simulink model "compare"  (R2015a)
settings: Solver=ode45  StartTime=0.0  StopTime=10.0  RelTol=1e-3
InitFcn:
  | %% DSPBuilder Start
  | alt_dspbuilder_update_model(bdroot)
  | %% DSPBuilder End
libraries: allblocks_alteradspbuilder2 x801
(part 1 of 9)
settings Model: Creator=ASUS  LastModifiedBy=ASUS

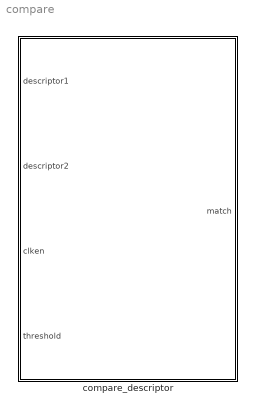
== system compare ==
  compare_descriptor : Subsystem

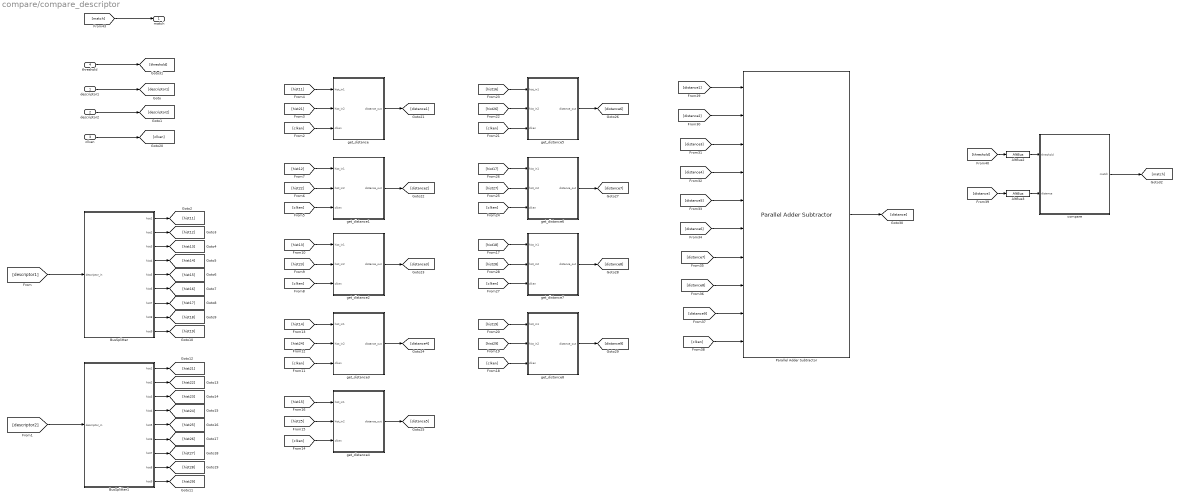
== system compare/compare_descriptor ==
  descriptor1 : Inport
  descriptor2 : Inport  Port=2
  clken : Inport  Port=3
  threshold : Inport  Port=4
  AltBus2 : allblocks_alteradspbuilder2/AltBus  BusType=Unsigned Integer  bwl=16  bwr=0  saturate=off  floatingPointInput=on  floatingPointOutput=on  logOutputs=off  logFile=C:\Users\ASUS\Desktop\final_sift_fpga\tb_compare\compare_compare%5Fdescriptor_AltBus2.fixedpointlog
  AltBus3 : allblocks_alteradspbuilder2/AltBus  BusType=Unsigned Integer  bwl=16  bwr=0  saturate=off  floatingPointInput=on  floatingPointOutput=on  logOutputs=off  logFile=C:\Users\ASUS\Desktop\final_sift_fpga\tb_compare\compare_compare%5Fdescriptor_AltBus3.fixedpointlog
  BusSplitter : Subsystem
  BusSplitter1 : Subsystem
  Parallel Adder Subtractor : allblocks_alteradspbuilder2/Parallel Adder Subtractor  number_of_inputs=9  direction=+  use_pipeline=on  pipeline_display=4  phase_selection=1  use_ena=on  use_aclr=off  allowFloatingPointOverride=on  logOutputs=off  logFile=C:\Users\ASUS\Desktop\final_sift_fpga\tb_compare\compare_compare%5Fdescriptor_Parallel+Adder+Subtractor.fixedpointlog
  compare : Subsystem
  get_distance : Subsystem
  get_distance1 : Subsystem
  get_distance2 : Subsystem
  get_distance3 : Subsystem
  get_distance4 : Subsystem
  get_distance5 : Subsystem
  get_distance6 : Subsystem
  get_distance7 : Subsystem
  get_distance8 : Subsystem
  match : Outport
  wires:
  descriptor1/1 -> [descriptor1]
  descriptor2/1 -> [descriptor2]
  [descriptor1] -> BusSplitter/1(descriptor_in)
  [descriptor2] -> BusSplitter1/1(descriptor_in)
  BusSplitter/1(hist1) -> [hist11]
  BusSplitter/2(hist2) -> [hist12]
  BusSplitter/3(hist3) -> [hist13]
  BusSplitter/4(hist4) -> [hist14]
  BusSplitter/5(hist5) -> [hist15]
  BusSplitter/6(hist6) -> [hist16]
  BusSplitter/7(hist7) -> [hist17]
  BusSplitter/8(hist8) -> [hist18]
  BusSplitter/9(hist9) -> [hist19]
  BusSplitter1/1(hist1) -> [hist21]
  BusSplitter1/2(hist2) -> [hist22]
  BusSplitter1/3(hist3) -> [hist23]
  BusSplitter1/4(hist4) -> [hist24]
  BusSplitter1/5(hist5) -> [hist25]
  BusSplitter1/6(hist6) -> [hist26]
  BusSplitter1/7(hist7) -> [hist27]
  BusSplitter1/8(hist8) -> [hist28]
  BusSplitter1/9(hist9) -> [hist29]
  clken/1 -> [clken]
  [clken] -> get_distance/3(clken)
  [hist21] -> get_distance/2(hist_in2)
  [hist11] -> get_distance/1(hist_in1)
  get_distance/1(distance_out) -> [distance1]
  [clken] -> get_distance1/3(clken)
  [hist22] -> get_distance1/2(hist_in2)
  [hist12] -> get_distance1/1(hist_in1)
  get_distance1/1(distance_out) -> [distance2]
  [clken] -> get_distance2/3(clken)
  [hist23] -> get_distance2/2(hist_in2)
  [hist13] -> get_distance2/1(hist_in1)
  get_distance2/1(distance_out) -> [distance3]
  [clken] -> get_distance3/3(clken)
  [hist24] -> get_distance3/2(hist_in2)
  [hist14] -> get_distance3/1(hist_in1)
  get_distance3/1(distance_out) -> [distance4]
  [clken] -> get_distance4/3(clken)
  [hist25] -> get_distance4/2(hist_in2)
  [hist15] -> get_distance4/1(hist_in1)
  get_distance4/1(distance_out) -> [distance5]
  [clken] -> get_distance5/3(clken)
  [hist26] -> get_distance5/2(hist_in2)
  [hist16] -> get_distance5/1(hist_in1)
  get_distance5/1(distance_out) -> [distance6]
  [clken] -> get_distance6/3(clken)
  [hist27] -> get_distance6/2(hist_in2)
  [hist17] -> get_distance6/1(hist_in1)
  get_distance6/1(distance_out) -> [distance7]
  [clken] -> get_distance7/3(clken)
  [hist28] -> get_distance7/2(hist_in2)
  [hist18] -> get_distance7/1(hist_in1)
  get_distance7/1(distance_out) -> [distance8]
  [clken] -> get_distance8/3(clken)
  [hist29] -> get_distance8/2(hist_in2)
  [hist19] -> get_distance8/1(hist_in1)
  get_distance8/1(distance_out) -> [distance9]
  [distance1] -> Parallel Adder Subtractor/1
  [distance2] -> Parallel Adder Subtractor/2
  [distance3] -> Parallel Adder Subtractor/3
  [distance4] -> Parallel Adder Subtractor/4
  [distance5] -> Parallel Adder Subtractor/5
  [distance6] -> Parallel Adder Subtractor/6
  [distance7] -> Parallel Adder Subtractor/7
  [distance8] -> Parallel Adder Subtractor/8
  [distance9] -> Parallel Adder Subtractor/9
  [clken] -> Parallel Adder Subtractor/10
  threshold/1 -> [threshold]
  [distance] -> AltBus3/1
  [threshold] -> AltBus2/1
  [match] -> match/1
  compare/1(match) -> [match]
  Parallel Adder Subtractor/1 -> [distance]
  AltBus2/1 -> compare/1(threshold)
  AltBus3/1 -> compare/2(distance)

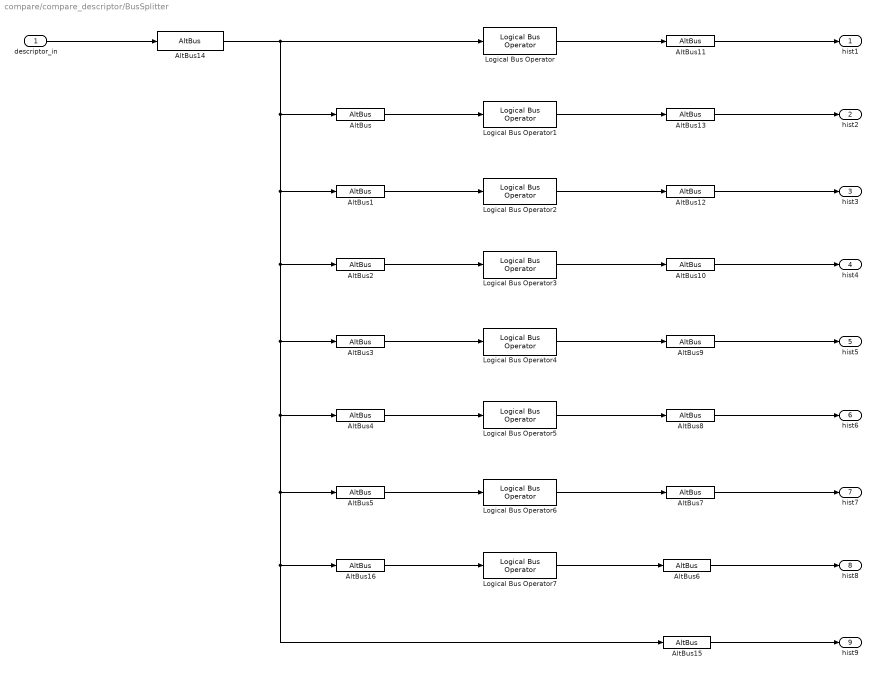
== system compare/compare_descriptor/BusSplitter ==
  descriptor_in : Inport
  AltBus : allblocks_alteradspbuilder2/AltBus  BusType=Unsigned Integer  bwl=1024  bwr=0  saturate=off  floatingPointInput=on  floatingPointOutput=on  logOutputs=off  logFile=C:\Users\ASUS\Desktop\sift_fpga\Octave_2\tb_test_final_sift\test%5Ffinal%5Fsift_sift%5Foctave1_matching_compare%5Fdescriptor_BusSplitter_AltBus.fixedpointlog
  AltBus1 : allblocks_alteradspbuilder2/AltBus  BusType=Unsigned Integer  bwl=896  bwr=0  saturate=off  floatingPointInput=on  floatingPointOutput=on  logOutputs=off  logFile=C:\Users\ASUS\Desktop\sift_fpga\Octave_2\tb_test_final_sift\test%5Ffinal%5Fsift_sift%5Foctave1_matching_compare%5Fdescriptor_BusSplitter_AltBus1.fixedpointlog
  AltBus10 : allblocks_alteradspbuilder2/AltBus  BusType=Unsigned Integer  bwl=128  bwr=0  saturate=off  floatingPointInput=on  floatingPointOutput=on  logOutputs=off  logFile=C:\Users\ASUS\Desktop\sift_fpga\Octave_2\tb_test_final_sift\test%5Ffinal%5Fsift_sift%5Foctave1_matching_compare%5Fdescriptor_BusSplitter_AltBus10.fixedpointlog
  AltBus11 : allblocks_alteradspbuilder2/AltBus  BusType=Unsigned Integer  bwl=128  bwr=0  saturate=off  floatingPointInput=on  floatingPointOutput=on  logOutputs=off  logFile=C:\Users\ASUS\Desktop\sift_fpga\Octave_2\tb_test_final_sift\test%5Ffinal%5Fsift_sift%5Foctave1_matching_compare%5Fdescriptor_BusSplitter_AltBus11.fixedpointlog
  AltBus12 : allblocks_alteradspbuilder2/AltBus  BusType=Unsigned Integer  bwl=128  bwr=0  saturate=off  floatingPointInput=on  floatingPointOutput=on  logOutputs=off  logFile=C:\Users\ASUS\Desktop\sift_fpga\Octave_2\tb_test_final_sift\test%5Ffinal%5Fsift_sift%5Foctave1_matching_compare%5Fdescriptor_BusSplitter_AltBus12.fixedpointlog
  AltBus13 : allblocks_alteradspbuilder2/AltBus  BusType=Unsigned Integer  bwl=128  bwr=0  saturate=off  floatingPointInput=on  floatingPointOutput=on  logOutputs=off  logFile=C:\Users\ASUS\Desktop\sift_fpga\Octave_2\tb_test_final_sift\test%5Ffinal%5Fsift_sift%5Foctave1_matching_compare%5Fdescriptor_BusSplitter_AltBus13.fixedpointlog
  AltBus14 : allblocks_alteradspbuilder2/AltBus  BusType=Unsigned Integer  bwl=16*8*9  bwr=0  saturate=off  floatingPointInput=on  floatingPointOutput=on  logOutputs=off  logFile=C:\Users\ASUS\Desktop\sift_fpga\Octave_2\tb_test_final_sift\test%5Ffinal%5Fsift_sift%5Foctave1_matching_compare%5Fdescriptor_BusSplitter_AltBus14.fixedpointlog
  AltBus15 : allblocks_alteradspbuilder2/AltBus  BusType=Unsigned Integer  bwl=128  bwr=0  saturate=off  floatingPointInput=on  floatingPointOutput=on  logOutputs=off  logFile=C:\Users\ASUS\Desktop\sift_fpga\Octave_2\tb_test_final_sift\test%5Ffinal%5Fsift_sift%5Foctave1_matching_compare%5Fdescriptor_BusSplitter_AltBus15.fixedpointlog
  AltBus16 : allblocks_alteradspbuilder2/AltBus  BusType=Unsigned Integer  bwl=256  bwr=0  saturate=off  floatingPointInput=on  floatingPointOutput=on  logOutputs=off  logFile=C:\Users\ASUS\Desktop\sift_fpga\Octave_2\tb_test_final_sift\test%5Ffinal%5Fsift_sift%5Foctave1_matching_compare%5Fdescriptor_BusSplitter_AltBus16.fixedpointlog
  AltBus2 : allblocks_alteradspbuilder2/AltBus  BusType=Unsigned Integer  bwl=768  bwr=0  saturate=off  floatingPointInput=on  floatingPointOutput=on  logOutputs=off  logFile=C:\Users\ASUS\Desktop\sift_fpga\Octave_2\tb_test_final_sift\test%5Ffinal%5Fsift_sift%5Foctave1_matching_compare%5Fdescriptor_BusSplitter_AltBus2.fixedpointlog
  AltBus3 : allblocks_alteradspbuilder2/AltBus  BusType=Unsigned Integer  bwl=640  bwr=0  saturate=off  floatingPointInput=on  floatingPointOutput=on  logOutputs=off  logFile=C:\Users\ASUS\Desktop\sift_fpga\Octave_2\tb_test_final_sift\test%5Ffinal%5Fsift_sift%5Foctave1_matching_compare%5Fdescriptor_BusSplitter_AltBus3.fixedpointlog
  AltBus4 : allblocks_alteradspbuilder2/AltBus  BusType=Unsigned Integer  bwl=512  bwr=0  saturate=off  floatingPointInput=on  floatingPointOutput=on  logOutputs=off  logFile=C:\Users\ASUS\Desktop\sift_fpga\Octave_2\tb_test_final_sift\test%5Ffinal%5Fsift_sift%5Foctave1_matching_compare%5Fdescriptor_BusSplitter_AltBus4.fixedpointlog
  AltBus5 : allblocks_alteradspbuilder2/AltBus  BusType=Unsigned Integer  bwl=384  bwr=0  saturate=off  floatingPointInput=on  floatingPointOutput=on  logOutputs=off  logFile=C:\Users\ASUS\Desktop\sift_fpga\Octave_2\tb_test_final_sift\test%5Ffinal%5Fsift_sift%5Foctave1_matching_compare%5Fdescriptor_BusSplitter_AltBus5.fixedpointlog
  AltBus6 : allblocks_alteradspbuilder2/AltBus  BusType=Unsigned Integer  bwl=128  bwr=0  saturate=off  floatingPointInput=on  floatingPointOutput=on  logOutputs=off  logFile=C:\Users\ASUS\Desktop\sift_fpga\Octave_2\tb_test_final_sift\test%5Ffinal%5Fsift_sift%5Foctave1_matching_compare%5Fdescriptor_BusSplitter_AltBus6.fixedpointlog
  AltBus7 : allblocks_alteradspbuilder2/AltBus  BusType=Unsigned Integer  bwl=128  bwr=0  saturate=off  floatingPointInput=on  floatingPointOutput=on  logOutputs=off  logFile=C:\Users\ASUS\Desktop\sift_fpga\Octave_2\tb_test_final_sift\test%5Ffinal%5Fsift_sift%5Foctave1_matching_compare%5Fdescriptor_BusSplitter_AltBus7.fixedpointlog
  AltBus8 : allblocks_alteradspbuilder2/AltBus  BusType=Unsigned Integer  bwl=128  bwr=0  saturate=off  floatingPointInput=on  floatingPointOutput=on  logOutputs=off  logFile=C:\Users\ASUS\Desktop\sift_fpga\Octave_2\tb_test_final_sift\test%5Ffinal%5Fsift_sift%5Foctave1_matching_compare%5Fdescriptor_BusSplitter_AltBus8.fixedpointlog
  AltBus9 : allblocks_alteradspbuilder2/AltBus  BusType=Unsigned Integer  bwl=128  bwr=0  saturate=off  floatingPointInput=on  floatingPointOutput=on  logOutputs=off  logFile=C:\Users\ASUS\Desktop\sift_fpga\Octave_2\tb_test_final_sift\test%5Ffinal%5Fsift_sift%5Foctave1_matching_compare%5Fdescriptor_BusSplitter_AltBus9.fixedpointlog
  Logical Bus Operator : allblocks_alteradspbuilder2/Logical Bus Operator  BusType=Unsigned Integer  bwl=1152  bwr=0  LogicalOp_text=Shift Right  mask_value_num=-5  shift_amount=8*128  force_sign_ext=off  pipeline_display=0
  Logical Bus Operator1 : allblocks_alteradspbuilder2/Logical Bus Operator  BusType=Unsigned Integer  bwl=1024  bwr=0  LogicalOp_text=Shift Right  mask_value_num=-5  shift_amount=7*128  force_sign_ext=off  pipeline_display=0
  Logical Bus Operator2 : allblocks_alteradspbuilder2/Logical Bus Operator  BusType=Unsigned Integer  bwl=896  bwr=0  LogicalOp_text=Shift Right  mask_value_num=-5  shift_amount=6*128  force_sign_ext=off  pipeline_display=0
  Logical Bus Operator3 : allblocks_alteradspbuilder2/Logical Bus Operator  BusType=Unsigned Integer  bwl=768  bwr=0  LogicalOp_text=Shift Right  mask_value_num=-5  shift_amount=5*128  force_sign_ext=off  pipeline_display=0
  Logical Bus Operator4 : allblocks_alteradspbuilder2/Logical Bus Operator  BusType=Unsigned Integer  bwl=640  bwr=0  LogicalOp_text=Shift Right  mask_value_num=-5  shift_amount=4*128  force_sign_ext=off  pipeline_display=0
  Logical Bus Operator5 : allblocks_alteradspbuilder2/Logical Bus Operator  BusType=Unsigned Integer  bwl=512  bwr=0  LogicalOp_text=Shift Right  mask_value_num=-5  shift_amount=3*128  force_sign_ext=off  pipeline_display=0
  Logical Bus Operator6 : allblocks_alteradspbuilder2/Logical Bus Operator  BusType=Unsigned Integer  bwl=384  bwr=0  LogicalOp_text=Shift Right  mask_value_num=-5  shift_amount=2*128  force_sign_ext=off  pipeline_display=0
  Logical Bus Operator7 : allblocks_alteradspbuilder2/Logical Bus Operator  BusType=Unsigned Integer  bwl=256  bwr=0  LogicalOp_text=Shift Right  mask_value_num=-5  shift_amount=128  force_sign_ext=off  pipeline_display=0
  hist1 : Outport
  hist2 : Outport  Port=2
  hist3 : Outport  Port=3
  hist4 : Outport  Port=4
  hist5 : Outport  Port=5
  hist6 : Outport  Port=6
  hist7 : Outport  Port=7
  hist8 : Outport  Port=8
  hist9 : Outport  Port=9
  wires:
  Logical Bus Operator6/1 -> AltBus7/1
  AltBus1/1 -> Logical Bus Operator2/1
  AltBus9/1 -> hist5/1
  AltBus8/1 -> hist6/1
  AltBus7/1 -> hist7/1
  AltBus6/1 -> hist8/1
  AltBus/1 -> Logical Bus Operator1/1
  AltBus10/1 -> hist4/1
  AltBus12/1 -> hist3/1
  AltBus11/1 -> hist1/1
  AltBus3/1 -> Logical Bus Operator4/1
  AltBus2/1 -> Logical Bus Operator3/1
  AltBus4/1 -> Logical Bus Operator5/1
  descriptor_in/1 -> AltBus14/1
  AltBus5/1 -> Logical Bus Operator6/1
  Logical Bus Operator1/1 -> AltBus13/1
  Logical Bus Operator2/1 -> AltBus12/1
  Logical Bus Operator/1 -> AltBus11/1
  Logical Bus Operator5/1 -> AltBus8/1
  Logical Bus Operator4/1 -> AltBus9/1
  Logical Bus Operator3/1 -> AltBus10/1
  AltBus13/1 -> hist2/1
  AltBus15/1 -> hist9/1
  AltBus14/1 -> AltBus15/1, AltBus16/1, AltBus5/1, AltBus4/1, AltBus3/1, AltBus2/1, AltBus1/1, AltBus/1, Logical Bus Operator/1
  AltBus16/1 -> Logical Bus Operator7/1
  Logical Bus Operator7/1 -> AltBus6/1

== system compare/compare_descriptor/BusSplitter1 ==
  descriptor_in : Inport
  AltBus : allblocks_alteradspbuilder2/AltBus  BusType=Unsigned Integer  bwl=1024  bwr=0  saturate=off  floatingPointInput=on  floatingPointOutput=on  logOutputs=off  logFile=C:\Users\ASUS\Desktop\sift_fpga\Octave_2\tb_test_final_sift\test%5Ffinal%5Fsift_sift%5Foctave1_matching_compare%5Fdescriptor_BusSplitter1_AltBus.fixedpointlog
  AltBus1 : allblocks_alteradspbuilder2/AltBus  BusType=Unsigned Integer  bwl=896  bwr=0  saturate=off  floatingPointInput=on  floatingPointOutput=on  logOutputs=off  logFile=C:\Users\ASUS\Desktop\sift_fpga\Octave_2\tb_test_final_sift\test%5Ffinal%5Fsift_sift%5Foctave1_matching_compare%5Fdescriptor_BusSplitter1_AltBus1.fixedpointlog
  AltBus10 : allblocks_alteradspbuilder2/AltBus  BusType=Unsigned Integer  bwl=128  bwr=0  saturate=off  floatingPointInput=on  floatingPointOutput=on  logOutputs=off  logFile=C:\Users\ASUS\Desktop\sift_fpga\Octave_2\tb_test_final_sift\test%5Ffinal%5Fsift_sift%5Foctave1_matching_compare%5Fdescriptor_BusSplitter1_AltBus10.fixedpointlog
  AltBus11 : allblocks_alteradspbuilder2/AltBus  BusType=Unsigned Integer  bwl=128  bwr=0  saturate=off  floatingPointInput=on  floatingPointOutput=on  logOutputs=off  logFile=C:\Users\ASUS\Desktop\sift_fpga\Octave_2\tb_test_final_sift\test%5Ffinal%5Fsift_sift%5Foctave1_matching_compare%5Fdescriptor_BusSplitter1_AltBus11.fixedpointlog
  AltBus12 : allblocks_alteradspbuilder2/AltBus  BusType=Unsigned Integer  bwl=128  bwr=0  saturate=off  floatingPointInput=on  floatingPointOutput=on  logOutputs=off  logFile=C:\Users\ASUS\Desktop\sift_fpga\Octave_2\tb_test_final_sift\test%5Ffinal%5Fsift_sift%5Foctave1_matching_compare%5Fdescriptor_BusSplitter1_AltBus12.fixedpointlog
  AltBus13 : allblocks_alteradspbuilder2/AltBus  BusType=Unsigned Integer  bwl=128  bwr=0  saturate=off  floatingPointInput=on  floatingPointOutput=on  logOutputs=off  logFile=C:\Users\ASUS\Desktop\sift_fpga\Octave_2\tb_test_final_sift\test%5Ffinal%5Fsift_sift%5Foctave1_matching_compare%5Fdescriptor_BusSplitter1_AltBus13.fixedpointlog
  AltBus14 : allblocks_alteradspbuilder2/AltBus  BusType=Unsigned Integer  bwl=16*8*9  bwr=0  saturate=off  floatingPointInput=on  floatingPointOutput=on  logOutputs=off  logFile=C:\Users\ASUS\Desktop\sift_fpga\Octave_2\tb_test_final_sift\test%5Ffinal%5Fsift_sift%5Foctave1_matching_compare%5Fdescriptor_BusSplitter1_AltBus14.fixedpointlog
  AltBus15 : allblocks_alteradspbuilder2/AltBus  BusType=Unsigned Integer  bwl=128  bwr=0  saturate=off  floatingPointInput=on  floatingPointOutput=on  logOutputs=off  logFile=C:\Users\ASUS\Desktop\sift_fpga\Octave_2\tb_test_final_sift\test%5Ffinal%5Fsift_sift%5Foctave1_matching_compare%5Fdescriptor_BusSplitter1_AltBus15.fixedpointlog
  AltBus16 : allblocks_alteradspbuilder2/AltBus  BusType=Unsigned Integer  bwl=256  bwr=0  saturate=off  floatingPointInput=on  floatingPointOutput=on  logOutputs=off  logFile=C:\Users\ASUS\Desktop\sift_fpga\Octave_2\tb_test_final_sift\test%5Ffinal%5Fsift_sift%5Foctave1_matching_compare%5Fdescriptor_BusSplitter1_AltBus16.fixedpointlog
  AltBus2 : allblocks_alteradspbuilder2/AltBus  BusType=Unsigned Integer  bwl=768  bwr=0  saturate=off  floatingPointInput=on  floatingPointOutput=on  logOutputs=off  logFile=C:\Users\ASUS\Desktop\sift_fpga\Octave_2\tb_test_final_sift\test%5Ffinal%5Fsift_sift%5Foctave1_matching_compare%5Fdescriptor_BusSplitter1_AltBus2.fixedpointlog
  AltBus3 : allblocks_alteradspbuilder2/AltBus  BusType=Unsigned Integer  bwl=640  bwr=0  saturate=off  floatingPointInput=on  floatingPointOutput=on  logOutputs=off  logFile=C:\Users\ASUS\Desktop\sift_fpga\Octave_2\tb_test_final_sift\test%5Ffinal%5Fsift_sift%5Foctave1_matching_compare%5Fdescriptor_BusSplitter1_AltBus3.fixedpointlog
  AltBus4 : allblocks_alteradspbuilder2/AltBus  BusType=Unsigned Integer  bwl=512  bwr=0  saturate=off  floatingPointInput=on  floatingPointOutput=on  logOutputs=off  logFile=C:\Users\ASUS\Desktop\sift_fpga\Octave_2\tb_test_final_sift\test%5Ffinal%5Fsift_sift%5Foctave1_matching_compare%5Fdescriptor_BusSplitter1_AltBus4.fixedpointlog
  AltBus5 : allblocks_alteradspbuilder2/AltBus  BusType=Unsigned Integer  bwl=384  bwr=0  saturate=off  floatingPointInput=on  floatingPointOutput=on  logOutputs=off  logFile=C:\Users\ASUS\Desktop\sift_fpga\Octave_2\tb_test_final_sift\test%5Ffinal%5Fsift_sift%5Foctave1_matching_compare%5Fdescriptor_BusSplitter1_AltBus5.fixedpointlog
  AltBus6 : allblocks_alteradspbuilder2/AltBus  BusType=Unsigned Integer  bwl=128  bwr=0  saturate=off  floatingPointInput=on  floatingPointOutput=on  logOutputs=off  logFile=C:\Users\ASUS\Desktop\sift_fpga\Octave_2\tb_test_final_sift\test%5Ffinal%5Fsift_sift%5Foctave1_matching_compare%5Fdescriptor_BusSplitter1_AltBus6.fixedpointlog
  AltBus7 : allblocks_alteradspbuilder2/AltBus  BusType=Unsigned Integer  bwl=128  bwr=0  saturate=off  floatingPointInput=on  floatingPointOutput=on  logOutputs=off  logFile=C:\Users\ASUS\Desktop\sift_fpga\Octave_2\tb_test_final_sift\test%5Ffinal%5Fsift_sift%5Foctave1_matching_compare%5Fdescriptor_BusSplitter1_AltBus7.fixedpointlog
  AltBus8 : allblocks_alteradspbuilder2/AltBus  BusType=Unsigned Integer  bwl=128  bwr=0  saturate=off  floatingPointInput=on  floatingPointOutput=on  logOutputs=off  logFile=C:\Users\ASUS\Desktop\sift_fpga\Octave_2\tb_test_final_sift\test%5Ffinal%5Fsift_sift%5Foctave1_matching_compare%5Fdescriptor_BusSplitter1_AltBus8.fixedpointlog
  AltBus9 : allblocks_alteradspbuilder2/AltBus  BusType=Unsigned Integer  bwl=128  bwr=0  saturate=off  floatingPointInput=on  floatingPointOutput=on  logOutputs=off  logFile=C:\Users\ASUS\Desktop\sift_fpga\Octave_2\tb_test_final_sift\test%5Ffinal%5Fsift_sift%5Foctave1_matching_compare%5Fdescriptor_BusSplitter1_AltBus9.fixedpointlog
  Logical Bus Operator : allblocks_alteradspbuilder2/Logical Bus Operator  BusType=Unsigned Integer  bwl=1152  bwr=0  LogicalOp_text=Shift Right  mask_value_num=-5  shift_amount=8*128  force_sign_ext=off  pipeline_display=0
  Logical Bus Operator1 : allblocks_alteradspbuilder2/Logical Bus Operator  BusType=Unsigned Integer  bwl=1024  bwr=0  LogicalOp_text=Shift Right  mask_value_num=-5  shift_amount=7*128  force_sign_ext=off  pipeline_display=0
  Logical Bus Operator2 : allblocks_alteradspbuilder2/Logical Bus Operator  BusType=Unsigned Integer  bwl=896  bwr=0  LogicalOp_text=Shift Right  mask_value_num=-5  shift_amount=6*128  force_sign_ext=off  pipeline_display=0
  Logical Bus Operator3 : allblocks_alteradspbuilder2/Logical Bus Operator  BusType=Unsigned Integer  bwl=768  bwr=0  LogicalOp_text=Shift Right  mask_value_num=-5  shift_amount=5*128  force_sign_ext=off  pipeline_display=0
  Logical Bus Operator4 : allblocks_alteradspbuilder2/Logical Bus Operator  BusType=Unsigned Integer  bwl=640  bwr=0  LogicalOp_text=Shift Right  mask_value_num=-5  shift_amount=4*128  force_sign_ext=off  pipeline_display=0
  Logical Bus Operator5 : allblocks_alteradspbuilder2/Logical Bus Operator  BusType=Unsigned Integer  bwl=512  bwr=0  LogicalOp_text=Shift Right  mask_value_num=-5  shift_amount=3*128  force_sign_ext=off  pipeline_display=0
  Logical Bus Operator6 : allblocks_alteradspbuilder2/Logical Bus Operator  BusType=Unsigned Integer  bwl=384  bwr=0  LogicalOp_text=Shift Right  mask_value_num=-5  shift_amount=2*128  force_sign_ext=off  pipeline_display=0
  Logical Bus Operator7 : allblocks_alteradspbuilder2/Logical Bus Operator  BusType=Unsigned Integer  bwl=256  bwr=0  LogicalOp_text=Shift Right  mask_value_num=-5  shift_amount=128  force_sign_ext=off  pipeline_display=0
  hist1 : Outport
  hist2 : Outport  Port=2
  hist3 : Outport  Port=3
  hist4 : Outport  Port=4
  hist5 : Outport  Port=5
  hist6 : Outport  Port=6
  hist7 : Outport  Port=7
  hist8 : Outport  Port=8
  hist9 : Outport  Port=9
  wires:
  Logical Bus Operator6/1 -> AltBus7/1
  AltBus1/1 -> Logical Bus Operator2/1
  AltBus9/1 -> hist5/1
  AltBus8/1 -> hist6/1
  AltBus7/1 -> hist7/1
  AltBus6/1 -> hist8/1
  AltBus/1 -> Logical Bus Operator1/1
  AltBus10/1 -> hist4/1
  AltBus12/1 -> hist3/1
  AltBus11/1 -> hist1/1
  AltBus3/1 -> Logical Bus Operator4/1
  AltBus2/1 -> Logical Bus Operator3/1
  AltBus4/1 -> Logical Bus Operator5/1
  descriptor_in/1 -> AltBus14/1
  AltBus5/1 -> Logical Bus Operator6/1
  Logical Bus Operator1/1 -> AltBus13/1
  Logical Bus Operator2/1 -> AltBus12/1
  Logical Bus Operator/1 -> AltBus11/1
  Logical Bus Operator5/1 -> AltBus8/1
  Logical Bus Operator4/1 -> AltBus9/1
  Logical Bus Operator3/1 -> AltBus10/1
  AltBus13/1 -> hist2/1
  AltBus15/1 -> hist9/1
  AltBus14/1 -> AltBus15/1, AltBus16/1, AltBus5/1, AltBus4/1, AltBus3/1, AltBus2/1, AltBus1/1, AltBus/1, Logical Bus Operator/1
  AltBus16/1 -> Logical Bus Operator7/1
  Logical Bus Operator7/1 -> AltBus6/1

== system compare/compare_descriptor/compare ==
  threshold : Inport
  distance : Inport  Port=2
  Comparator : allblocks_alteradspbuilder2/Comparator  direction=a > b  pipeline_display=0  allowFloatingPointOverride=on  logOutputs=off  logFile=C:\Users\ASUS\Desktop\sift_fpga\Octave_2\tb_test_final_sift\test%5Ffinal%5Fsift_sift%5Foctave1_matching_compare%5Fdescriptor_compare_Comparator.fixedpointlog
  match : Outport
  wires:
  threshold/1 -> [threshold]
  distance/1 -> [distance]
  [match] -> match/1
  [threshold] -> Comparator/1
  [distance] -> Comparator/2
  Comparator/1 -> [match]

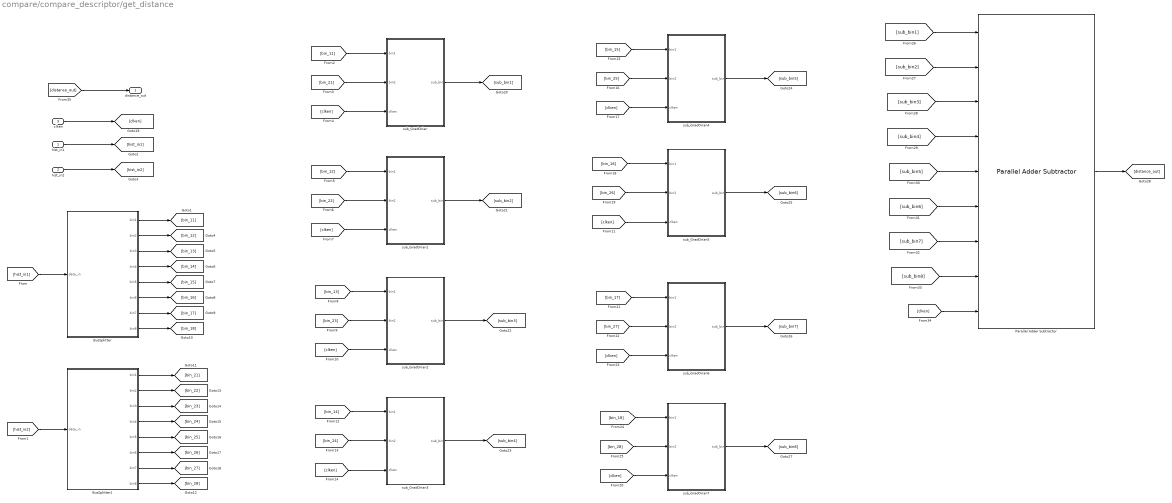
== system compare/compare_descriptor/get_distance ==
  hist_in1 : Inport
  hist_in2 : Inport  Port=2
  clken : Inport  Port=3
  BusSplitter : Subsystem
  BusSplitter1 : Subsystem
  Parallel Adder Subtractor : allblocks_alteradspbuilder2/Parallel Adder Subtractor  number_of_inputs=8  direction=+  use_pipeline=on  pipeline_display=3  phase_selection=1  use_ena=on  use_aclr=off  allowFloatingPointOverride=on  logOutputs=off  logFile=C:\Users\ASUS\Desktop\sift_fpga\Octave_2\tb_test_final_sift\test%5Ffinal%5Fsift_sift%5Foctave1_matching_compare%5Fdescriptor_get%5Fdistance_Parallel+Adder+Subtractor.fixedpointlog
  sub_GradOrian : Subsystem
  sub_GradOrian1 : Subsystem
  sub_GradOrian2 : Subsystem
  sub_GradOrian3 : Subsystem
  sub_GradOrian4 : Subsystem
  sub_GradOrian5 : Subsystem
  sub_GradOrian6 : Subsystem
  sub_GradOrian7 : Subsystem
  distance_out : Outport
  wires:
  hist_in2/1 -> [hist_in2]
  hist_in1/1 -> [hist_in1]
  [hist_in1] -> BusSplitter/1(data_in)
  [hist_in2] -> BusSplitter1/1(data_in)
  BusSplitter/1(bin1) -> [bin_11]
  BusSplitter/2(bin2) -> [bin_12]
  BusSplitter/3(bin3) -> [bin_13]
  BusSplitter/4(bin4) -> [bin_14]
  BusSplitter/5(bin5) -> [bin_15]
  BusSplitter/6(bin6) -> [bin_16]
  BusSplitter/7(bin7) -> [bin_17]
  BusSplitter/8(bin8) -> [bin_18]
  BusSplitter1/1(bin1) -> [bin_21]
  BusSplitter1/2(bin2) -> [bin_22]
  BusSplitter1/3(bin3) -> [bin_23]
  BusSplitter1/4(bin4) -> [bin_24]
  BusSplitter1/5(bin5) -> [bin_25]
  BusSplitter1/6(bin6) -> [bin_26]
  BusSplitter1/7(bin7) -> [bin_27]
  BusSplitter1/8(bin8) -> [bin_28]
  [bin_21] -> sub_GradOrian/2(bin2)
  [bin_11] -> sub_GradOrian/1(bin1)
  clken/1 -> [clken]
  [clken] -> sub_GradOrian/3(clken)
  sub_GradOrian/1(sub_bin) -> [sub_bin1]
  [bin_22] -> sub_GradOrian1/2(bin2)
  [bin_12] -> sub_GradOrian1/1(bin1)
  [clken] -> sub_GradOrian1/3(clken)
  sub_GradOrian1/1(sub_bin) -> [sub_bin2]
  [bin_23] -> sub_GradOrian2/2(bin2)
  [bin_13] -> sub_GradOrian2/1(bin1)
  [clken] -> sub_GradOrian2/3(clken)
  sub_GradOrian2/1(sub_bin) -> [sub_bin3]
  [bin_24] -> sub_GradOrian3/2(bin2)
  [bin_14] -> sub_GradOrian3/1(bin1)
  [clken] -> sub_GradOrian3/3(clken)
  sub_GradOrian3/1(sub_bin) -> [sub_bin4]
  [bin_25] -> sub_GradOrian4/2(bin2)
  [bin_15] -> sub_GradOrian4/1(bin1)
  [clken] -> sub_GradOrian4/3(clken)
  sub_GradOrian4/1(sub_bin) -> [sub_bin5]
  [bin_26] -> sub_GradOrian5/2(bin2)
  [bin_16] -> sub_GradOrian5/1(bin1)
  [clken] -> sub_GradOrian5/3(clken)
  sub_GradOrian5/1(sub_bin) -> [sub_bin6]
  [bin_27] -> sub_GradOrian6/2(bin2)
  [bin_17] -> sub_GradOrian6/1(bin1)
  [clken] -> sub_GradOrian6/3(clken)
  sub_GradOrian6/1(sub_bin) -> [sub_bin7]
  [bin_28] -> sub_GradOrian7/2(bin2)
  [bin_18] -> sub_GradOrian7/1(bin1)
  [clken] -> sub_GradOrian7/3(clken)
  sub_GradOrian7/1(sub_bin) -> [sub_bin8]
  [sub_bin1] -> Parallel Adder Subtractor/1
  [sub_bin2] -> Parallel Adder Subtractor/2
  [sub_bin3] -> Parallel Adder Subtractor/3
  [sub_bin4] -> Parallel Adder Subtractor/4
  [sub_bin5] -> Parallel Adder Subtractor/5
  [sub_bin6] -> Parallel Adder Subtractor/6
  [sub_bin7] -> Parallel Adder Subtractor/7
  [sub_bin8] -> Parallel Adder Subtractor/8
  [clken] -> Parallel Adder Subtractor/9
  Parallel Adder Subtractor/1 -> [distance_out]
  [distance_out] -> distance_out/1

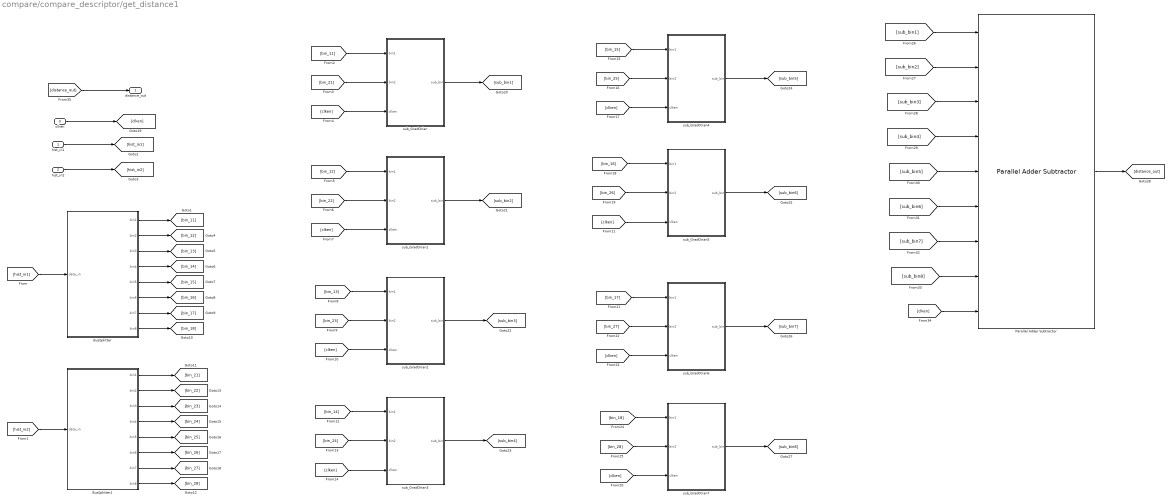
== system compare/compare_descriptor/get_distance1 ==
  hist_in1 : Inport
  hist_in2 : Inport  Port=2
  clken : Inport  Port=3
  BusSplitter : Subsystem
  BusSplitter1 : Subsystem
  Parallel Adder Subtractor : allblocks_alteradspbuilder2/Parallel Adder Subtractor  number_of_inputs=8  direction=+  use_pipeline=on  pipeline_display=3  phase_selection=1  use_ena=on  use_aclr=off  allowFloatingPointOverride=on  logOutputs=off  logFile=C:\Users\ASUS\Desktop\sift_fpga\Octave_2\tb_test_final_sift\test%5Ffinal%5Fsift_sift%5Foctave1_matching_compare%5Fdescriptor_get%5Fdistance1_Parallel+Adder+Subtractor.fixedpointlog
  sub_GradOrian : Subsystem
  sub_GradOrian1 : Subsystem
  sub_GradOrian2 : Subsystem
  sub_GradOrian3 : Subsystem
  sub_GradOrian4 : Subsystem
  sub_GradOrian5 : Subsystem
  sub_GradOrian6 : Subsystem
  sub_GradOrian7 : Subsystem
  distance_out : Outport
  wires:
  hist_in2/1 -> [hist_in2]
  hist_in1/1 -> [hist_in1]
  [hist_in1] -> BusSplitter/1(data_in)
  [hist_in2] -> BusSplitter1/1(data_in)
  BusSplitter/1(bin1) -> [bin_11]
  BusSplitter/2(bin2) -> [bin_12]
  BusSplitter/3(bin3) -> [bin_13]
  BusSplitter/4(bin4) -> [bin_14]
  BusSplitter/5(bin5) -> [bin_15]
  BusSplitter/6(bin6) -> [bin_16]
  BusSplitter/7(bin7) -> [bin_17]
  BusSplitter/8(bin8) -> [bin_18]
  BusSplitter1/1(bin1) -> [bin_21]
  BusSplitter1/2(bin2) -> [bin_22]
  BusSplitter1/3(bin3) -> [bin_23]
  BusSplitter1/4(bin4) -> [bin_24]
  BusSplitter1/5(bin5) -> [bin_25]
  BusSplitter1/6(bin6) -> [bin_26]
  BusSplitter1/7(bin7) -> [bin_27]
  BusSplitter1/8(bin8) -> [bin_28]
  [bin_21] -> sub_GradOrian/2(bin2)
  [bin_11] -> sub_GradOrian/1(bin1)
  clken/1 -> [clken]
  [clken] -> sub_GradOrian/3(clken)
  sub_GradOrian/1(sub_bin) -> [sub_bin1]
  [bin_22] -> sub_GradOrian1/2(bin2)
  [bin_12] -> sub_GradOrian1/1(bin1)
  [clken] -> sub_GradOrian1/3(clken)
  sub_GradOrian1/1(sub_bin) -> [sub_bin2]
  [bin_23] -> sub_GradOrian2/2(bin2)
  [bin_13] -> sub_GradOrian2/1(bin1)
  [clken] -> sub_GradOrian2/3(clken)
  sub_GradOrian2/1(sub_bin) -> [sub_bin3]
  [bin_24] -> sub_GradOrian3/2(bin2)
  [bin_14] -> sub_GradOrian3/1(bin1)
  [clken] -> sub_GradOrian3/3(clken)
  sub_GradOrian3/1(sub_bin) -> [sub_bin4]
  [bin_25] -> sub_GradOrian4/2(bin2)
  [bin_15] -> sub_GradOrian4/1(bin1)
  [clken] -> sub_GradOrian4/3(clken)
  sub_GradOrian4/1(sub_bin) -> [sub_bin5]
  [bin_26] -> sub_GradOrian5/2(bin2)
  [bin_16] -> sub_GradOrian5/1(bin1)
  [clken] -> sub_GradOrian5/3(clken)
  sub_GradOrian5/1(sub_bin) -> [sub_bin6]
  [bin_27] -> sub_GradOrian6/2(bin2)
  [bin_17] -> sub_GradOrian6/1(bin1)
  [clken] -> sub_GradOrian6/3(clken)
  sub_GradOrian6/1(sub_bin) -> [sub_bin7]
  [bin_28] -> sub_GradOrian7/2(bin2)
  [bin_18] -> sub_GradOrian7/1(bin1)
  [clken] -> sub_GradOrian7/3(clken)
  sub_GradOrian7/1(sub_bin) -> [sub_bin8]
  [sub_bin1] -> Parallel Adder Subtractor/1
  [sub_bin2] -> Parallel Adder Subtractor/2
  [sub_bin3] -> Parallel Adder Subtractor/3
  [sub_bin4] -> Parallel Adder Subtractor/4
  [sub_bin5] -> Parallel Adder Subtractor/5
  [sub_bin6] -> Parallel Adder Subtractor/6
  [sub_bin7] -> Parallel Adder Subtractor/7
  [sub_bin8] -> Parallel Adder Subtractor/8
  [clken] -> Parallel Adder Subtractor/9
  Parallel Adder Subtractor/1 -> [distance_out]
  [distance_out] -> distance_out/1

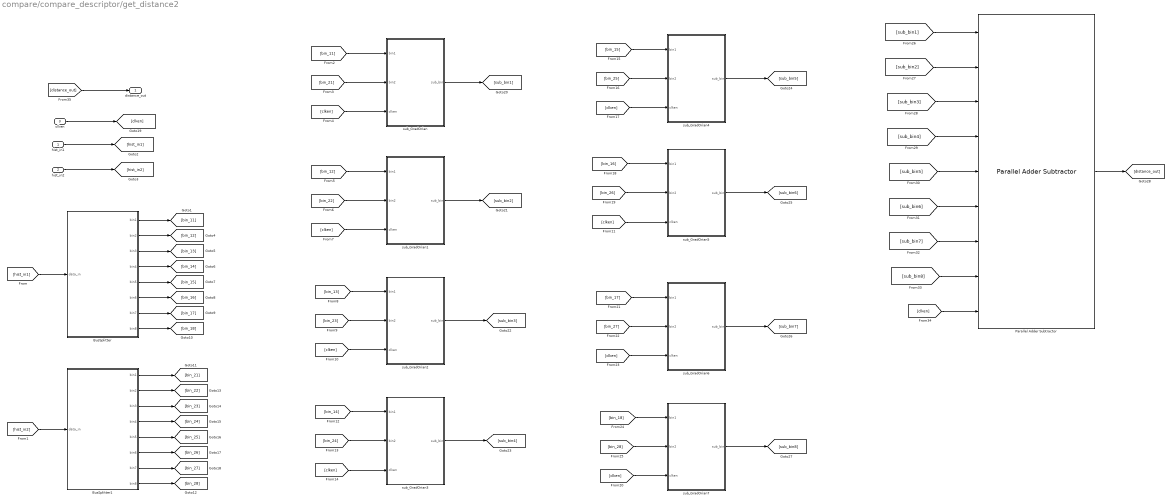
== system compare/compare_descriptor/get_distance2 ==
  hist_in1 : Inport
  hist_in2 : Inport  Port=2
  clken : Inport  Port=3
  BusSplitter : Subsystem
  BusSplitter1 : Subsystem
  Parallel Adder Subtractor : allblocks_alteradspbuilder2/Parallel Adder Subtractor  number_of_inputs=8  direction=+  use_pipeline=on  pipeline_display=3  phase_selection=1  use_ena=on  use_aclr=off  allowFloatingPointOverride=on  logOutputs=off  logFile=C:\Users\ASUS\Desktop\sift_fpga\Octave_2\tb_test_final_sift\test%5Ffinal%5Fsift_sift%5Foctave1_matching_compare%5Fdescriptor_get%5Fdistance2_Parallel+Adder+Subtractor.fixedpointlog
  sub_GradOrian : Subsystem
  sub_GradOrian1 : Subsystem
  sub_GradOrian2 : Subsystem
  sub_GradOrian3 : Subsystem
  sub_GradOrian4 : Subsystem
  sub_GradOrian5 : Subsystem
  sub_GradOrian6 : Subsystem
  sub_GradOrian7 : Subsystem
  distance_out : Outport
  wires:
  hist_in2/1 -> [hist_in2]
  hist_in1/1 -> [hist_in1]
  [hist_in1] -> BusSplitter/1(data_in)
  [hist_in2] -> BusSplitter1/1(data_in)
  BusSplitter/1(bin1) -> [bin_11]
  BusSplitter/2(bin2) -> [bin_12]
  BusSplitter/3(bin3) -> [bin_13]
  BusSplitter/4(bin4) -> [bin_14]
  BusSplitter/5(bin5) -> [bin_15]
  BusSplitter/6(bin6) -> [bin_16]
  BusSplitter/7(bin7) -> [bin_17]
  BusSplitter/8(bin8) -> [bin_18]
  BusSplitter1/1(bin1) -> [bin_21]
  BusSplitter1/2(bin2) -> [bin_22]
  BusSplitter1/3(bin3) -> [bin_23]
  BusSplitter1/4(bin4) -> [bin_24]
  BusSplitter1/5(bin5) -> [bin_25]
  BusSplitter1/6(bin6) -> [bin_26]
  BusSplitter1/7(bin7) -> [bin_27]
  BusSplitter1/8(bin8) -> [bin_28]
  [bin_21] -> sub_GradOrian/2(bin2)
  [bin_11] -> sub_GradOrian/1(bin1)
  clken/1 -> [clken]
  [clken] -> sub_GradOrian/3(clken)
  sub_GradOrian/1(sub_bin) -> [sub_bin1]
  [bin_22] -> sub_GradOrian1/2(bin2)
  [bin_12] -> sub_GradOrian1/1(bin1)
  [clken] -> sub_GradOrian1/3(clken)
  sub_GradOrian1/1(sub_bin) -> [sub_bin2]
  [bin_23] -> sub_GradOrian2/2(bin2)
  [bin_13] -> sub_GradOrian2/1(bin1)
  [clken] -> sub_GradOrian2/3(clken)
  sub_GradOrian2/1(sub_bin) -> [sub_bin3]
  [bin_24] -> sub_GradOrian3/2(bin2)
  [bin_14] -> sub_GradOrian3/1(bin1)
  [clken] -> sub_GradOrian3/3(clken)
  sub_GradOrian3/1(sub_bin) -> [sub_bin4]
  [bin_25] -> sub_GradOrian4/2(bin2)
  [bin_15] -> sub_GradOrian4/1(bin1)
  [clken] -> sub_GradOrian4/3(clken)
  sub_GradOrian4/1(sub_bin) -> [sub_bin5]
  [bin_26] -> sub_GradOrian5/2(bin2)
  [bin_16] -> sub_GradOrian5/1(bin1)
  [clken] -> sub_GradOrian5/3(clken)
  sub_GradOrian5/1(sub_bin) -> [sub_bin6]
  [bin_27] -> sub_GradOrian6/2(bin2)
  [bin_17] -> sub_GradOrian6/1(bin1)
  [clken] -> sub_GradOrian6/3(clken)
  sub_GradOrian6/1(sub_bin) -> [sub_bin7]
  [bin_28] -> sub_GradOrian7/2(bin2)
  [bin_18] -> sub_GradOrian7/1(bin1)
  [clken] -> sub_GradOrian7/3(clken)
  sub_GradOrian7/1(sub_bin) -> [sub_bin8]
  [sub_bin1] -> Parallel Adder Subtractor/1
  [sub_bin2] -> Parallel Adder Subtractor/2
  [sub_bin3] -> Parallel Adder Subtractor/3
  [sub_bin4] -> Parallel Adder Subtractor/4
  [sub_bin5] -> Parallel Adder Subtractor/5
  [sub_bin6] -> Parallel Adder Subtractor/6
  [sub_bin7] -> Parallel Adder Subtractor/7
  [sub_bin8] -> Parallel Adder Subtractor/8
  [clken] -> Parallel Adder Subtractor/9
  Parallel Adder Subtractor/1 -> [distance_out]
  [distance_out] -> distance_out/1

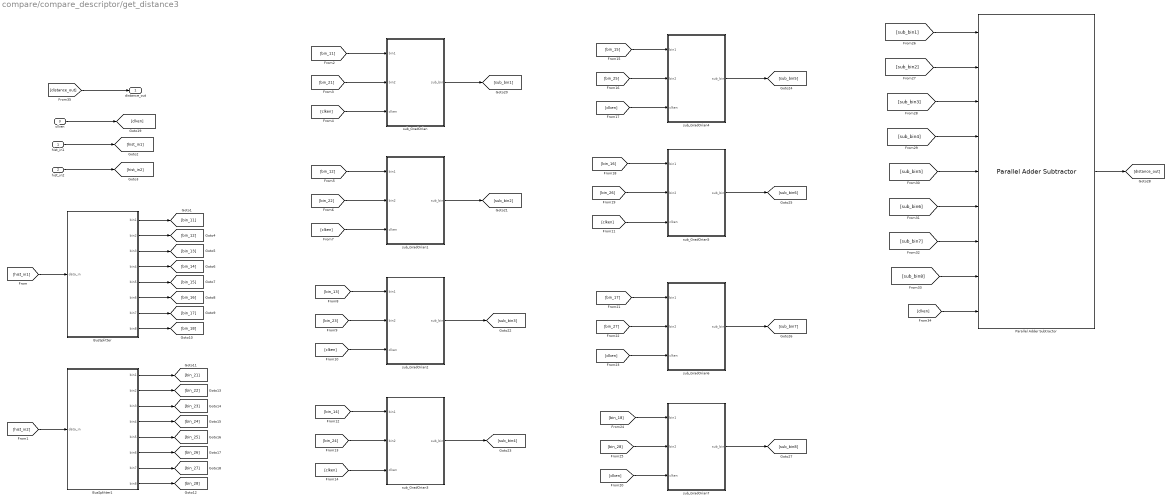
== system compare/compare_descriptor/get_distance3 ==
  hist_in1 : Inport
  hist_in2 : Inport  Port=2
  clken : Inport  Port=3
  BusSplitter : Subsystem
  BusSplitter1 : Subsystem
  Parallel Adder Subtractor : allblocks_alteradspbuilder2/Parallel Adder Subtractor  number_of_inputs=8  direction=+  use_pipeline=on  pipeline_display=3  phase_selection=1  use_ena=on  use_aclr=off  allowFloatingPointOverride=on  logOutputs=off  logFile=C:\Users\ASUS\Desktop\sift_fpga\Octave_2\tb_test_final_sift\test%5Ffinal%5Fsift_sift%5Foctave1_matching_compare%5Fdescriptor_get%5Fdistance3_Parallel+Adder+Subtractor.fixedpointlog
  sub_GradOrian : Subsystem
  sub_GradOrian1 : Subsystem
  sub_GradOrian2 : Subsystem
  sub_GradOrian3 : Subsystem
  sub_GradOrian4 : Subsystem
  sub_GradOrian5 : Subsystem
  sub_GradOrian6 : Subsystem
  sub_GradOrian7 : Subsystem
  distance_out : Outport
  wires:
  hist_in2/1 -> [hist_in2]
  hist_in1/1 -> [hist_in1]
  [hist_in1] -> BusSplitter/1(data_in)
  [hist_in2] -> BusSplitter1/1(data_in)
  BusSplitter/1(bin1) -> [bin_11]
  BusSplitter/2(bin2) -> [bin_12]
  BusSplitter/3(bin3) -> [bin_13]
  BusSplitter/4(bin4) -> [bin_14]
  BusSplitter/5(bin5) -> [bin_15]
  BusSplitter/6(bin6) -> [bin_16]
  BusSplitter/7(bin7) -> [bin_17]
  BusSplitter/8(bin8) -> [bin_18]
  BusSplitter1/1(bin1) -> [bin_21]
  BusSplitter1/2(bin2) -> [bin_22]
  BusSplitter1/3(bin3) -> [bin_23]
  BusSplitter1/4(bin4) -> [bin_24]
  BusSplitter1/5(bin5) -> [bin_25]
  BusSplitter1/6(bin6) -> [bin_26]
  BusSplitter1/7(bin7) -> [bin_27]
  BusSplitter1/8(bin8) -> [bin_28]
  [bin_21] -> sub_GradOrian/2(bin2)
  [bin_11] -> sub_GradOrian/1(bin1)
  clken/1 -> [clken]
  [clken] -> sub_GradOrian/3(clken)
  sub_GradOrian/1(sub_bin) -> [sub_bin1]
  [bin_22] -> sub_GradOrian1/2(bin2)
  [bin_12] -> sub_GradOrian1/1(bin1)
  [clken] -> sub_GradOrian1/3(clken)
  sub_GradOrian1/1(sub_bin) -> [sub_bin2]
  [bin_23] -> sub_GradOrian2/2(bin2)
  [bin_13] -> sub_GradOrian2/1(bin1)
  [clken] -> sub_GradOrian2/3(clken)
  sub_GradOrian2/1(sub_bin) -> [sub_bin3]
  [bin_24] -> sub_GradOrian3/2(bin2)
  [bin_14] -> sub_GradOrian3/1(bin1)
  [clken] -> sub_GradOrian3/3(clken)
  sub_GradOrian3/1(sub_bin) -> [sub_bin4]
  [bin_25] -> sub_GradOrian4/2(bin2)
  [bin_15] -> sub_GradOrian4/1(bin1)
  [clken] -> sub_GradOrian4/3(clken)
  sub_GradOrian4/1(sub_bin) -> [sub_bin5]
  [bin_26] -> sub_GradOrian5/2(bin2)
  [bin_16] -> sub_GradOrian5/1(bin1)
  [clken] -> sub_GradOrian5/3(clken)
  sub_GradOrian5/1(sub_bin) -> [sub_bin6]
  [bin_27] -> sub_GradOrian6/2(bin2)
  [bin_17] -> sub_GradOrian6/1(bin1)
  [clken] -> sub_GradOrian6/3(clken)
  sub_GradOrian6/1(sub_bin) -> [sub_bin7]
  [bin_28] -> sub_GradOrian7/2(bin2)
  [bin_18] -> sub_GradOrian7/1(bin1)
  [clken] -> sub_GradOrian7/3(clken)
  sub_GradOrian7/1(sub_bin) -> [sub_bin8]
  [sub_bin1] -> Parallel Adder Subtractor/1
  [sub_bin2] -> Parallel Adder Subtractor/2
  [sub_bin3] -> Parallel Adder Subtractor/3
  [sub_bin4] -> Parallel Adder Subtractor/4
  [sub_bin5] -> Parallel Adder Subtractor/5
  [sub_bin6] -> Parallel Adder Subtractor/6
  [sub_bin7] -> Parallel Adder Subtractor/7
  [sub_bin8] -> Parallel Adder Subtractor/8
  [clken] -> Parallel Adder Subtractor/9
  Parallel Adder Subtractor/1 -> [distance_out]
  [distance_out] -> distance_out/1

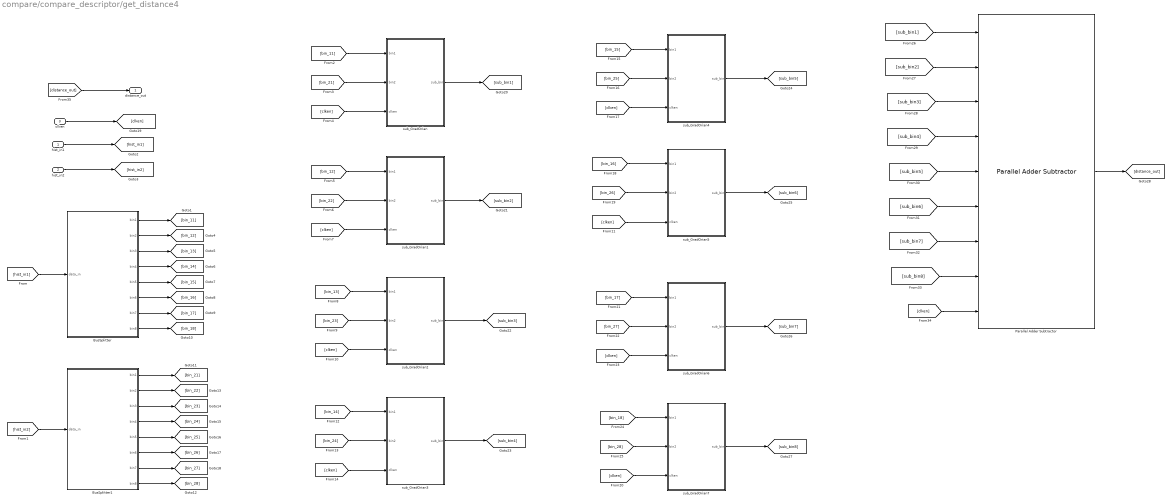
== system compare/compare_descriptor/get_distance4 ==
  hist_in1 : Inport
  hist_in2 : Inport  Port=2
  clken : Inport  Port=3
  BusSplitter : Subsystem
  BusSplitter1 : Subsystem
  Parallel Adder Subtractor : allblocks_alteradspbuilder2/Parallel Adder Subtractor  number_of_inputs=8  direction=+  use_pipeline=on  pipeline_display=3  phase_selection=1  use_ena=on  use_aclr=off  allowFloatingPointOverride=on  logOutputs=off  logFile=C:\Users\ASUS\Desktop\sift_fpga\Octave_2\tb_test_final_sift\test%5Ffinal%5Fsift_sift%5Foctave1_matching_compare%5Fdescriptor_get%5Fdistance4_Parallel+Adder+Subtractor.fixedpointlog
  sub_GradOrian : Subsystem
  sub_GradOrian1 : Subsystem
  sub_GradOrian2 : Subsystem
  sub_GradOrian3 : Subsystem
  sub_GradOrian4 : Subsystem
  sub_GradOrian5 : Subsystem
  sub_GradOrian6 : Subsystem
  sub_GradOrian7 : Subsystem
  distance_out : Outport
  wires:
  hist_in2/1 -> [hist_in2]
  hist_in1/1 -> [hist_in1]
  [hist_in1] -> BusSplitter/1(data_in)
  [hist_in2] -> BusSplitter1/1(data_in)
  BusSplitter/1(bin1) -> [bin_11]
  BusSplitter/2(bin2) -> [bin_12]
  BusSplitter/3(bin3) -> [bin_13]
  BusSplitter/4(bin4) -> [bin_14]
  BusSplitter/5(bin5) -> [bin_15]
  BusSplitter/6(bin6) -> [bin_16]
  BusSplitter/7(bin7) -> [bin_17]
  BusSplitter/8(bin8) -> [bin_18]
  BusSplitter1/1(bin1) -> [bin_21]
  BusSplitter1/2(bin2) -> [bin_22]
  BusSplitter1/3(bin3) -> [bin_23]
  BusSplitter1/4(bin4) -> [bin_24]
  BusSplitter1/5(bin5) -> [bin_25]
  BusSplitter1/6(bin6) -> [bin_26]
  BusSplitter1/7(bin7) -> [bin_27]
  BusSplitter1/8(bin8) -> [bin_28]
  [bin_21] -> sub_GradOrian/2(bin2)
  [bin_11] -> sub_GradOrian/1(bin1)
  clken/1 -> [clken]
  [clken] -> sub_GradOrian/3(clken)
  sub_GradOrian/1(sub_bin) -> [sub_bin1]
  [bin_22] -> sub_GradOrian1/2(bin2)
  [bin_12] -> sub_GradOrian1/1(bin1)
  [clken] -> sub_GradOrian1/3(clken)
  sub_GradOrian1/1(sub_bin) -> [sub_bin2]
  [bin_23] -> sub_GradOrian2/2(bin2)
  [bin_13] -> sub_GradOrian2/1(bin1)
  [clken] -> sub_GradOrian2/3(clken)
  sub_GradOrian2/1(sub_bin) -> [sub_bin3]
  [bin_24] -> sub_GradOrian3/2(bin2)
  [bin_14] -> sub_GradOrian3/1(bin1)
  [clken] -> sub_GradOrian3/3(clken)
  sub_GradOrian3/1(sub_bin) -> [sub_bin4]
  [bin_25] -> sub_GradOrian4/2(bin2)
  [bin_15] -> sub_GradOrian4/1(bin1)
  [clken] -> sub_GradOrian4/3(clken)
  sub_GradOrian4/1(sub_bin) -> [sub_bin5]
  [bin_26] -> sub_GradOrian5/2(bin2)
  [bin_16] -> sub_GradOrian5/1(bin1)
  [clken] -> sub_GradOrian5/3(clken)
  sub_GradOrian5/1(sub_bin) -> [sub_bin6]
  [bin_27] -> sub_GradOrian6/2(bin2)
  [bin_17] -> sub_GradOrian6/1(bin1)
  [clken] -> sub_GradOrian6/3(clken)
  sub_GradOrian6/1(sub_bin) -> [sub_bin7]
  [bin_28] -> sub_GradOrian7/2(bin2)
  [bin_18] -> sub_GradOrian7/1(bin1)
  [clken] -> sub_GradOrian7/3(clken)
  sub_GradOrian7/1(sub_bin) -> [sub_bin8]
  [sub_bin1] -> Parallel Adder Subtractor/1
  [sub_bin2] -> Parallel Adder Subtractor/2
  [sub_bin3] -> Parallel Adder Subtractor/3
  [sub_bin4] -> Parallel Adder Subtractor/4
  [sub_bin5] -> Parallel Adder Subtractor/5
  [sub_bin6] -> Parallel Adder Subtractor/6
  [sub_bin7] -> Parallel Adder Subtractor/7
  [sub_bin8] -> Parallel Adder Subtractor/8
  [clken] -> Parallel Adder Subtractor/9
  Parallel Adder Subtractor/1 -> [distance_out]
  [distance_out] -> distance_out/1

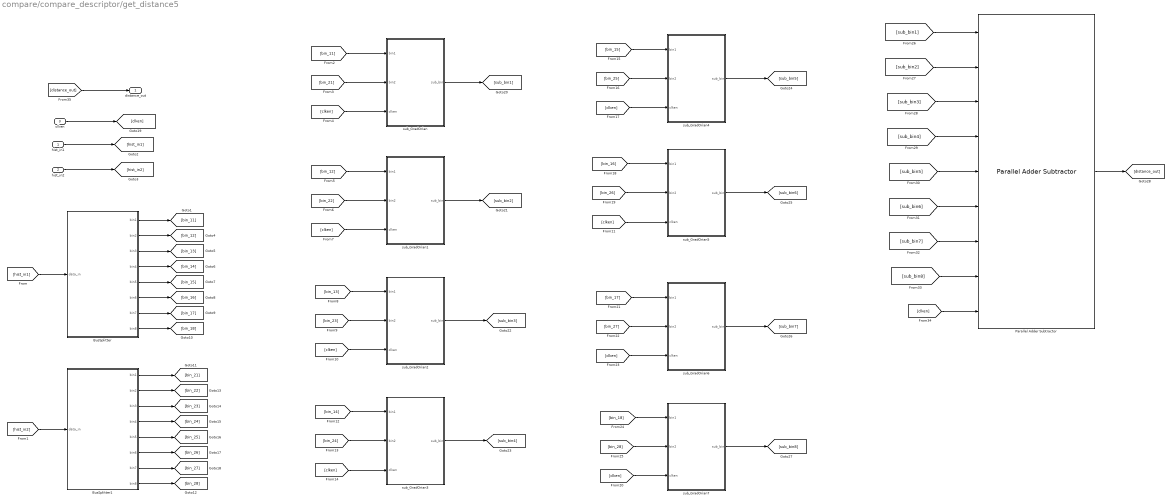
== system compare/compare_descriptor/get_distance5 ==
  hist_in1 : Inport
  hist_in2 : Inport  Port=2
  clken : Inport  Port=3
  BusSplitter : Subsystem
  BusSplitter1 : Subsystem
  Parallel Adder Subtractor : allblocks_alteradspbuilder2/Parallel Adder Subtractor  number_of_inputs=8  direction=+  use_pipeline=on  pipeline_display=3  phase_selection=1  use_ena=on  use_aclr=off  allowFloatingPointOverride=on  logOutputs=off  logFile=C:\Users\ASUS\Desktop\sift_fpga\Octave_2\tb_test_final_sift\test%5Ffinal%5Fsift_sift%5Foctave1_matching_compare%5Fdescriptor_get%5Fdistance5_Parallel+Adder+Subtractor.fixedpointlog
  sub_GradOrian : Subsystem
  sub_GradOrian1 : Subsystem
  sub_GradOrian2 : Subsystem
  sub_GradOrian3 : Subsystem
  sub_GradOrian4 : Subsystem
  sub_GradOrian5 : Subsystem
  sub_GradOrian6 : Subsystem
  sub_GradOrian7 : Subsystem
  distance_out : Outport
  wires:
  hist_in2/1 -> [hist_in2]
  hist_in1/1 -> [hist_in1]
  [hist_in1] -> BusSplitter/1(data_in)
  [hist_in2] -> BusSplitter1/1(data_in)
  BusSplitter/1(bin1) -> [bin_11]
  BusSplitter/2(bin2) -> [bin_12]
  BusSplitter/3(bin3) -> [bin_13]
  BusSplitter/4(bin4) -> [bin_14]
  BusSplitter/5(bin5) -> [bin_15]
  BusSplitter/6(bin6) -> [bin_16]
  BusSplitter/7(bin7) -> [bin_17]
  BusSplitter/8(bin8) -> [bin_18]
  BusSplitter1/1(bin1) -> [bin_21]
  BusSplitter1/2(bin2) -> [bin_22]
  BusSplitter1/3(bin3) -> [bin_23]
  BusSplitter1/4(bin4) -> [bin_24]
  BusSplitter1/5(bin5) -> [bin_25]
  BusSplitter1/6(bin6) -> [bin_26]
  BusSplitter1/7(bin7) -> [bin_27]
  BusSplitter1/8(bin8) -> [bin_28]
  [bin_21] -> sub_GradOrian/2(bin2)
  [bin_11] -> sub_GradOrian/1(bin1)
  clken/1 -> [clken]
  [clken] -> sub_GradOrian/3(clken)
  sub_GradOrian/1(sub_bin) -> [sub_bin1]
  [bin_22] -> sub_GradOrian1/2(bin2)
  [bin_12] -> sub_GradOrian1/1(bin1)
  [clken] -> sub_GradOrian1/3(clken)
  sub_GradOrian1/1(sub_bin) -> [sub_bin2]
  [bin_23] -> sub_GradOrian2/2(bin2)
  [bin_13] -> sub_GradOrian2/1(bin1)
  [clken] -> sub_GradOrian2/3(clken)
  sub_GradOrian2/1(sub_bin) -> [sub_bin3]
  [bin_24] -> sub_GradOrian3/2(bin2)
  [bin_14] -> sub_GradOrian3/1(bin1)
  [clken] -> sub_GradOrian3/3(clken)
  sub_GradOrian3/1(sub_bin) -> [sub_bin4]
  [bin_25] -> sub_GradOrian4/2(bin2)
  [bin_15] -> sub_GradOrian4/1(bin1)
  [clken] -> sub_GradOrian4/3(clken)
  sub_GradOrian4/1(sub_bin) -> [sub_bin5]
  [bin_26] -> sub_GradOrian5/2(bin2)
  [bin_16] -> sub_GradOrian5/1(bin1)
  [clken] -> sub_GradOrian5/3(clken)
  sub_GradOrian5/1(sub_bin) -> [sub_bin6]
  [bin_27] -> sub_GradOrian6/2(bin2)
  [bin_17] -> sub_GradOrian6/1(bin1)
  [clken] -> sub_GradOrian6/3(clken)
  sub_GradOrian6/1(sub_bin) -> [sub_bin7]
  [bin_28] -> sub_GradOrian7/2(bin2)
  [bin_18] -> sub_GradOrian7/1(bin1)
  [clken] -> sub_GradOrian7/3(clken)
  sub_GradOrian7/1(sub_bin) -> [sub_bin8]
  [sub_bin1] -> Parallel Adder Subtractor/1
  [sub_bin2] -> Parallel Adder Subtractor/2
  [sub_bin3] -> Parallel Adder Subtractor/3
  [sub_bin4] -> Parallel Adder Subtractor/4
  [sub_bin5] -> Parallel Adder Subtractor/5
  [sub_bin6] -> Parallel Adder Subtractor/6
  [sub_bin7] -> Parallel Adder Subtractor/7
  [sub_bin8] -> Parallel Adder Subtractor/8
  [clken] -> Parallel Adder Subtractor/9
  Parallel Adder Subtractor/1 -> [distance_out]
  [distance_out] -> distance_out/1

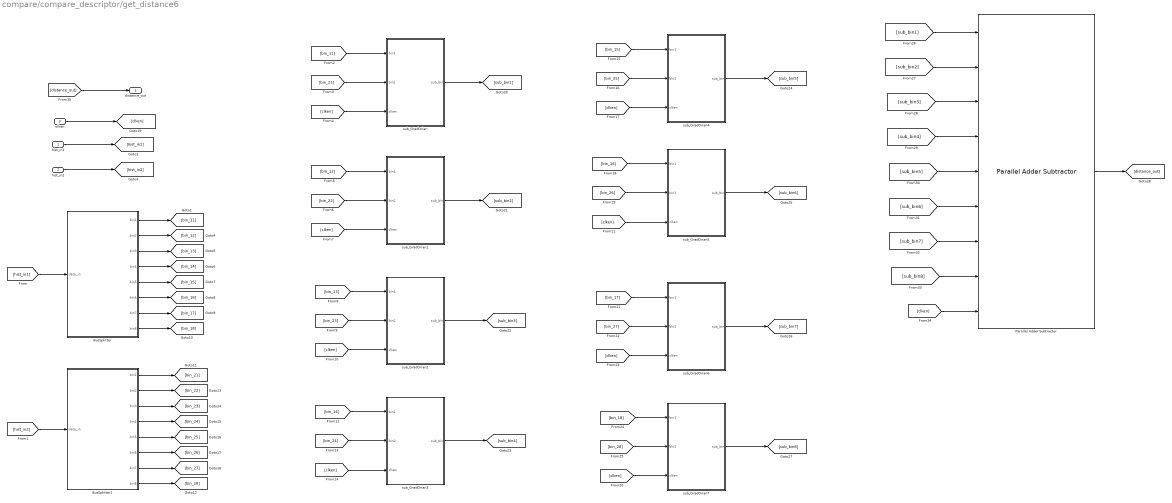
== system compare/compare_descriptor/get_distance6 ==
  hist_in1 : Inport
  hist_in2 : Inport  Port=2
  clken : Inport  Port=3
  BusSplitter : Subsystem
  BusSplitter1 : Subsystem
  Parallel Adder Subtractor : allblocks_alteradspbuilder2/Parallel Adder Subtractor  number_of_inputs=8  direction=+  use_pipeline=on  pipeline_display=3  phase_selection=1  use_ena=on  use_aclr=off  allowFloatingPointOverride=on  logOutputs=off  logFile=C:\Users\ASUS\Desktop\sift_fpga\Octave_2\tb_test_final_sift\test%5Ffinal%5Fsift_sift%5Foctave1_matching_compare%5Fdescriptor_get%5Fdistance6_Parallel+Adder+Subtractor.fixedpointlog
  sub_GradOrian : Subsystem
  sub_GradOrian1 : Subsystem
  sub_GradOrian2 : Subsystem
  sub_GradOrian3 : Subsystem
  sub_GradOrian4 : Subsystem
  sub_GradOrian5 : Subsystem
  sub_GradOrian6 : Subsystem
  sub_GradOrian7 : Subsystem
  distance_out : Outport
  wires:
  hist_in2/1 -> [hist_in2]
  hist_in1/1 -> [hist_in1]
  [hist_in1] -> BusSplitter/1(data_in)
  [hist_in2] -> BusSplitter1/1(data_in)
  BusSplitter/1(bin1) -> [bin_11]
  BusSplitter/2(bin2) -> [bin_12]
  BusSplitter/3(bin3) -> [bin_13]
  BusSplitter/4(bin4) -> [bin_14]
  BusSplitter/5(bin5) -> [bin_15]
  BusSplitter/6(bin6) -> [bin_16]
  BusSplitter/7(bin7) -> [bin_17]
  BusSplitter/8(bin8) -> [bin_18]
  BusSplitter1/1(bin1) -> [bin_21]
  BusSplitter1/2(bin2) -> [bin_22]
  BusSplitter1/3(bin3) -> [bin_23]
  BusSplitter1/4(bin4) -> [bin_24]
  BusSplitter1/5(bin5) -> [bin_25]
  BusSplitter1/6(bin6) -> [bin_26]
  BusSplitter1/7(bin7) -> [bin_27]
  BusSplitter1/8(bin8) -> [bin_28]
  [bin_21] -> sub_GradOrian/2(bin2)
  [bin_11] -> sub_GradOrian/1(bin1)
  clken/1 -> [clken]
  [clken] -> sub_GradOrian/3(clken)
  sub_GradOrian/1(sub_bin) -> [sub_bin1]
  [bin_22] -> sub_GradOrian1/2(bin2)
  [bin_12] -> sub_GradOrian1/1(bin1)
  [clken] -> sub_GradOrian1/3(clken)
  sub_GradOrian1/1(sub_bin) -> [sub_bin2]
  [bin_23] -> sub_GradOrian2/2(bin2)
  [bin_13] -> sub_GradOrian2/1(bin1)
  [clken] -> sub_GradOrian2/3(clken)
  sub_GradOrian2/1(sub_bin) -> [sub_bin3]
  [bin_24] -> sub_GradOrian3/2(bin2)
  [bin_14] -> sub_GradOrian3/1(bin1)
  [clken] -> sub_GradOrian3/3(clken)
  sub_GradOrian3/1(sub_bin) -> [sub_bin4]
  [bin_25] -> sub_GradOrian4/2(bin2)
  [bin_15] -> sub_GradOrian4/1(bin1)
  [clken] -> sub_GradOrian4/3(clken)
  sub_GradOrian4/1(sub_bin) -> [sub_bin5]
  [bin_26] -> sub_GradOrian5/2(bin2)
  [bin_16] -> sub_GradOrian5/1(bin1)
  [clken] -> sub_GradOrian5/3(clken)
  sub_GradOrian5/1(sub_bin) -> [sub_bin6]
  [bin_27] -> sub_GradOrian6/2(bin2)
  [bin_17] -> sub_GradOrian6/1(bin1)
  [clken] -> sub_GradOrian6/3(clken)
  sub_GradOrian6/1(sub_bin) -> [sub_bin7]
  [bin_28] -> sub_GradOrian7/2(bin2)
  [bin_18] -> sub_GradOrian7/1(bin1)
  [clken] -> sub_GradOrian7/3(clken)
  sub_GradOrian7/1(sub_bin) -> [sub_bin8]
  [sub_bin1] -> Parallel Adder Subtractor/1
  [sub_bin2] -> Parallel Adder Subtractor/2
  [sub_bin3] -> Parallel Adder Subtractor/3
  [sub_bin4] -> Parallel Adder Subtractor/4
  [sub_bin5] -> Parallel Adder Subtractor/5
  [sub_bin6] -> Parallel Adder Subtractor/6
  [sub_bin7] -> Parallel Adder Subtractor/7
  [sub_bin8] -> Parallel Adder Subtractor/8
  [clken] -> Parallel Adder Subtractor/9
  Parallel Adder Subtractor/1 -> [distance_out]
  [distance_out] -> distance_out/1

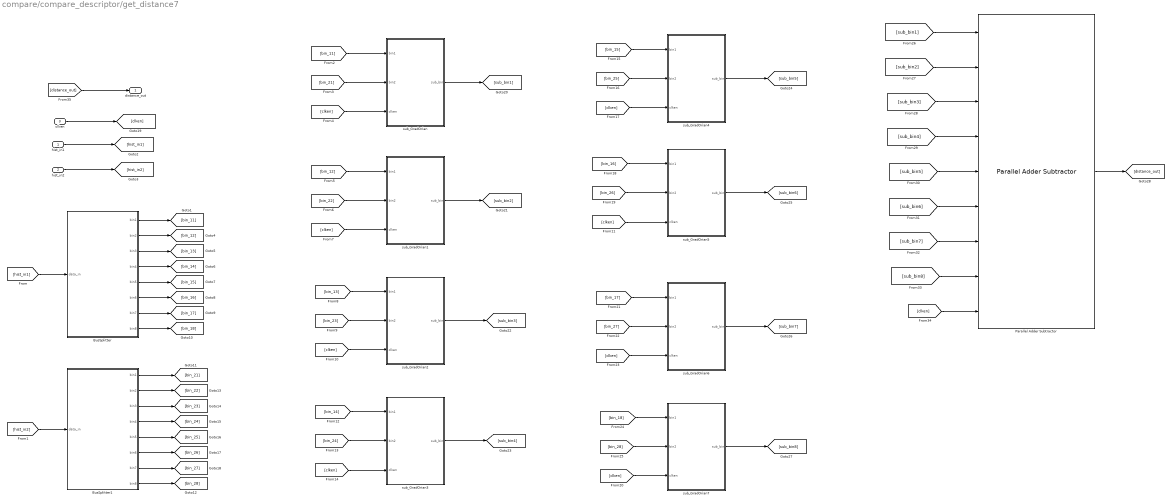
== system compare/compare_descriptor/get_distance7 ==
  hist_in1 : Inport
  hist_in2 : Inport  Port=2
  clken : Inport  Port=3
  BusSplitter : Subsystem
  BusSplitter1 : Subsystem
  Parallel Adder Subtractor : allblocks_alteradspbuilder2/Parallel Adder Subtractor  number_of_inputs=8  direction=+  use_pipeline=on  pipeline_display=3  phase_selection=1  use_ena=on  use_aclr=off  allowFloatingPointOverride=on  logOutputs=off  logFile=C:\Users\ASUS\Desktop\sift_fpga\Octave_2\tb_test_final_sift\test%5Ffinal%5Fsift_sift%5Foctave1_matching_compare%5Fdescriptor_get%5Fdistance7_Parallel+Adder+Subtractor.fixedpointlog
  sub_GradOrian : Subsystem
  sub_GradOrian1 : Subsystem
  sub_GradOrian2 : Subsystem
  sub_GradOrian3 : Subsystem
  sub_GradOrian4 : Subsystem
  sub_GradOrian5 : Subsystem
  sub_GradOrian6 : Subsystem
  sub_GradOrian7 : Subsystem
  distance_out : Outport
  wires:
  hist_in2/1 -> [hist_in2]
  hist_in1/1 -> [hist_in1]
  [hist_in1] -> BusSplitter/1(data_in)
  [hist_in2] -> BusSplitter1/1(data_in)
  BusSplitter/1(bin1) -> [bin_11]
  BusSplitter/2(bin2) -> [bin_12]
  BusSplitter/3(bin3) -> [bin_13]
  BusSplitter/4(bin4) -> [bin_14]
  BusSplitter/5(bin5) -> [bin_15]
  BusSplitter/6(bin6) -> [bin_16]
  BusSplitter/7(bin7) -> [bin_17]
  BusSplitter/8(bin8) -> [bin_18]
  BusSplitter1/1(bin1) -> [bin_21]
  BusSplitter1/2(bin2) -> [bin_22]
  BusSplitter1/3(bin3) -> [bin_23]
  BusSplitter1/4(bin4) -> [bin_24]
  BusSplitter1/5(bin5) -> [bin_25]
  BusSplitter1/6(bin6) -> [bin_26]
  BusSplitter1/7(bin7) -> [bin_27]
  BusSplitter1/8(bin8) -> [bin_28]
  [bin_21] -> sub_GradOrian/2(bin2)
  [bin_11] -> sub_GradOrian/1(bin1)
  clken/1 -> [clken]
  [clken] -> sub_GradOrian/3(clken)
  sub_GradOrian/1(sub_bin) -> [sub_bin1]
  [bin_22] -> sub_GradOrian1/2(bin2)
  [bin_12] -> sub_GradOrian1/1(bin1)
  [clken] -> sub_GradOrian1/3(clken)
  sub_GradOrian1/1(sub_bin) -> [sub_bin2]
  [bin_23] -> sub_GradOrian2/2(bin2)
  [bin_13] -> sub_GradOrian2/1(bin1)
  [clken] -> sub_GradOrian2/3(clken)
  sub_GradOrian2/1(sub_bin) -> [sub_bin3]
  [bin_24] -> sub_GradOrian3/2(bin2)
  [bin_14] -> sub_GradOrian3/1(bin1)
  [clken] -> sub_GradOrian3/3(clken)
  sub_GradOrian3/1(sub_bin) -> [sub_bin4]
  [bin_25] -> sub_GradOrian4/2(bin2)
  [bin_15] -> sub_GradOrian4/1(bin1)
  [clken] -> sub_GradOrian4/3(clken)
  sub_GradOrian4/1(sub_bin) -> [sub_bin5]
  [bin_26] -> sub_GradOrian5/2(bin2)
  [bin_16] -> sub_GradOrian5/1(bin1)
  [clken] -> sub_GradOrian5/3(clken)
  sub_GradOrian5/1(sub_bin) -> [sub_bin6]
  [bin_27] -> sub_GradOrian6/2(bin2)
  [bin_17] -> sub_GradOrian6/1(bin1)
  [clken] -> sub_GradOrian6/3(clken)
  sub_GradOrian6/1(sub_bin) -> [sub_bin7]
  [bin_28] -> sub_GradOrian7/2(bin2)
  [bin_18] -> sub_GradOrian7/1(bin1)
  [clken] -> sub_GradOrian7/3(clken)
  sub_GradOrian7/1(sub_bin) -> [sub_bin8]
  [sub_bin1] -> Parallel Adder Subtractor/1
  [sub_bin2] -> Parallel Adder Subtractor/2
  [sub_bin3] -> Parallel Adder Subtractor/3
  [sub_bin4] -> Parallel Adder Subtractor/4
  [sub_bin5] -> Parallel Adder Subtractor/5
  [sub_bin6] -> Parallel Adder Subtractor/6
  [sub_bin7] -> Parallel Adder Subtractor/7
  [sub_bin8] -> Parallel Adder Subtractor/8
  [clken] -> Parallel Adder Subtractor/9
  Parallel Adder Subtractor/1 -> [distance_out]
  [distance_out] -> distance_out/1
